simulink model "model"  (R2025a)
settings: Solver=VariableStepAuto  StartTime=0.0  StopTime=3000  RelTol=1e-3
libraries: dspadpt3 x1
settings Model: Creator=Mayur  LastModifiedBy=Mayur

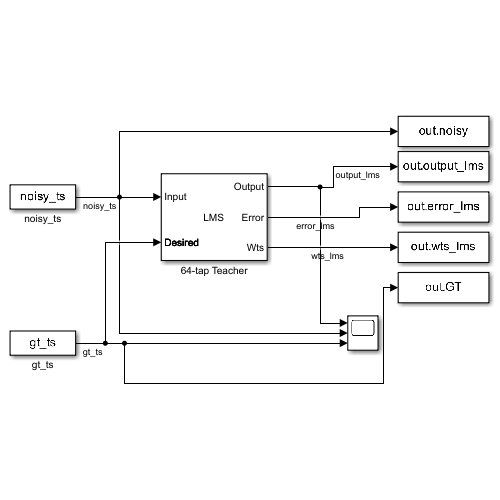
[thumbnail: Simulink's stored preview of the top-level diagram]
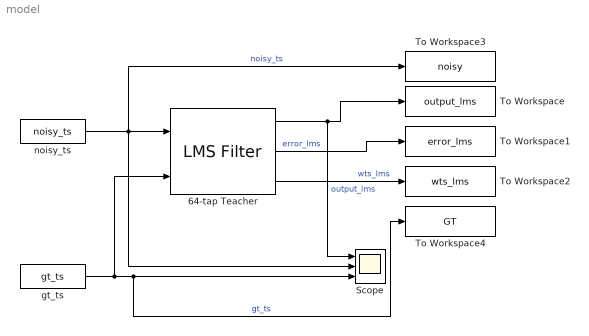
== system model ==
  64-tap Teacher : dspadpt3/LMS Filter  Algo=LMS  L=64  stepflag=Dialog  mu=0.5  leakage=1.0  ic=0  Adapt=off  resetflag=None  weights=on  addnparflag=off  roundingMode=Floor  overflowMode=off
  Scope : Scope  NumInputPorts=3
      settings: ActiveDisplayYMinimum=-0.28062009249258413  ActiveDisplayYMaximum=0.16766817604009
  To Workspace : ToWorkspace  VariableName=output_lms  SaveFormat=Timeseries  SampleTime=-1
  To Workspace1 : ToWorkspace  VariableName=error_lms  SaveFormat=Timeseries  SampleTime=-1
  To Workspace2 : ToWorkspace  VariableName=wts_lms  SaveFormat=Timeseries  SampleTime=-1
  To Workspace3 : ToWorkspace  VariableName=noisy  SaveFormat=Timeseries  SampleTime=-1
  To Workspace4 : ToWorkspace  VariableName=GT  SaveFormat=Timeseries  SampleTime=-1
  gt_ts : FromWorkspace  VariableName=gt_ts  SampleTime=1
  noisy_ts : FromWorkspace  VariableName=noisy_ts  SampleTime=1
  wires:
  64-tap Teacher/1 -> Scope/1, To Workspace/1  "output_lms"
  64-tap Teacher/2 -> To Workspace1/1  "error_lms"
  64-tap Teacher/3 -> To Workspace2/1  "wts_lms"
  noisy_ts/1 -> To Workspace3/1, 64-tap Teacher/1, Scope/2  "noisy_ts"
  gt_ts/1 -> 64-tap Teacher/2, To Workspace4/1, Scope/3  "gt_ts"
